simulink model "BKK7"  (Simulink 7.3)
settings: Solver=ode45  StartTime=0.0  StopTime=60  RelTol=1e-3
libraries: simulink x4
settings Model: Creator=AlexHomeLab  LastModifiedBy=Sainquake

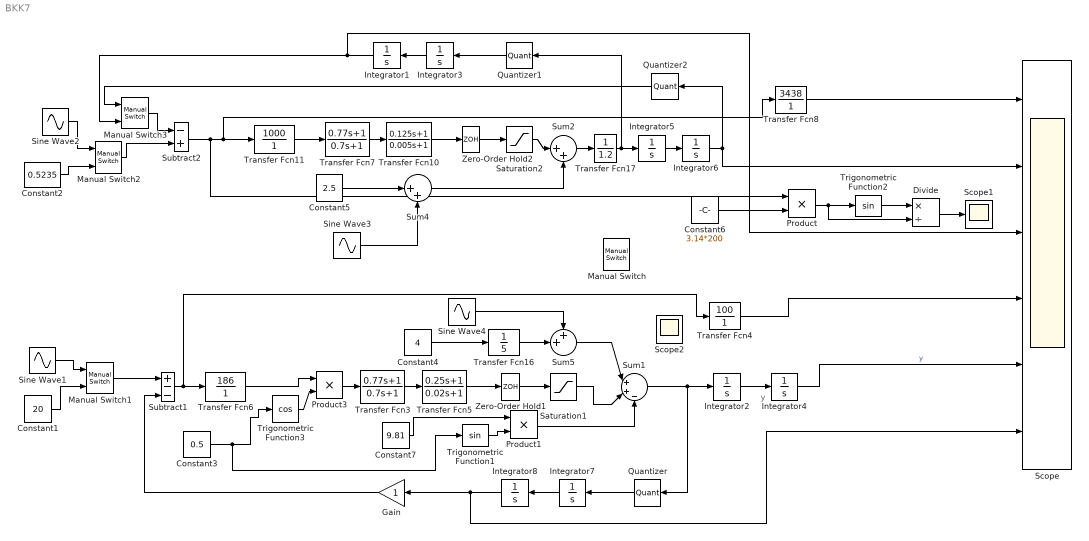
== system BKK7 ==
  note: y
  Constant1 : Constant  Value=20
  Constant2 : Constant  Value=0.5235
  Constant3 : Constant  Value=0.5
  Constant4 : Constant  Value=4
  Constant5 : Constant  Value=2.5
  Constant6 : Constant  Value=3.14*200
  Constant7 : Constant  Value=9.81
  Divide : Product  Inputs=*/  OutDataType=fixdt(1, 16)  OutScaling=2^-10
  Gain : Gain  ParameterDataType=fixdt(1, 16)  ParameterScaling=2^0  OutDataType=fixdt(1, 16)  OutScaling=2^0
  Integrator{1..8} (8 alike) : Integrator
  Manual Switch : simulink/Signal Routing/Manual Switch  SystemSampleTime=-1  sw=1  action=0  varsize=off
  Manual Switch1 : simulink/Signal Routing/Manual Switch  SystemSampleTime=-1  sw=0  action=0  varsize=off
  Manual Switch2 : simulink/Signal Routing/Manual Switch  SystemSampleTime=-1  sw=0  action=0  varsize=off
  Manual Switch3 : simulink/Signal Routing/Manual Switch  SystemSampleTime=-1  sw=0  action=0  varsize=off
  Product : Product  OutDataType=fixdt(1, 16)  OutScaling=2^0  RndMeth=Zero
  Product1 : Product  RndMeth=Zero
  Product3 : Product  RndMeth=Zero
  Quantizer : Quantizer  QuantizationInterval=0.00390625  SampleTime=1/200
  Quantizer1 : Quantizer  QuantizationInterval=0.00390625  SampleTime=1/200
  Quantizer2 : Quantizer  QuantizationInterval=0.00390625  SampleTime=1/200
  Saturation1 : Saturate  UpperLimit=17.2  LowerLimit=-17.2
  Saturation2 : Saturate  UpperLimit=20  LowerLimit=-20
  Scope : Scope  NumInputPorts=6
      settings: YMin=-45~0~-500~0~-750~0  YMax=5~60~2000~25~2000~0.7  MaxDataPoints=5000000
  Scope1 : Scope
      settings: SaveName=ScopeData2  MaxDataPoints=500000
  Scope2 : Scope
      settings: YMin=4.916  YMax=4.927  MaxDataPoints=500000
  Sine Wave1 : Sin  Amplitude=0.1  Bias=0  Frequency=0.628  Phase=0  Samples=10  SampleTime=0  Offset=0
  Sine Wave2 : Sin  Amplitude=0.1  Bias=0  Frequency=0.628  Phase=0  Samples=10  SampleTime=0  Offset=0
  Sine Wave3 : Sin  Amplitude=0.5  Bias=0  Frequency=6.28  Phase=1.57  Samples=10  SampleTime=0  Offset=0
  Sine Wave4 : Sin  Amplitude=0.3  Bias=0  Frequency=0.3  Phase=1.57  Samples=10  SampleTime=0  Offset=0
  Subtract1 : Sum  Inputs=+--
  Subtract2 : Sum  Inputs=-+
  Sum1 : Sum  Inputs=|++-
  Sum2 : Sum  Inputs=|++
  Sum4 : Sum  Inputs=|++
  Sum5 : Sum  Inputs=++|
  Transfer Fcn10 : TransferFcn  Numerator=[0.125 1]  Denominator="[0.005  1]"
  Transfer Fcn11 : TransferFcn  Numerator=1000  Denominator=[ 1 ]
  Transfer Fcn16 : TransferFcn  Denominator=[ 5 ]
  Transfer Fcn17 : TransferFcn  Denominator=[ 1.2 ]
  Transfer Fcn3 : TransferFcn  Numerator=[0.77 1]  Denominator="[0.7  1]"
  Transfer Fcn4 : TransferFcn  Numerator=[100]  Denominator=[ 1 ]
  Transfer Fcn5 : TransferFcn  Numerator=[0.25 1]  Denominator="[0.02  1]"
  Transfer Fcn6 : TransferFcn  Numerator=186  Denominator=[ 1 ]
  Transfer Fcn7 : TransferFcn  Numerator=[0.77 1]  Denominator="[0.7  1]"
  Transfer Fcn8 : TransferFcn  Numerator=[3438]  Denominator=[ 1 ]
  Trigonometric Function1 : Trigonometry
  Trigonometric Function2 : Trigonometry
  Trigonometric Function3 : Trigonometry  Operator=cos
  Zero-Order Hold1 : ZeroOrderHold  SampleTime=1/200
  Zero-Order Hold2 : ZeroOrderHold  SampleTime=1/200
  wires:
  Subtract1/1 -> Transfer Fcn6/1, Transfer Fcn4/1
  Transfer Fcn3/1 -> Transfer Fcn5/1
  Integrator2/1 -> Integrator4/1
  Constant1/1 -> Manual Switch1/2
  Product1/1 -> Sum1/3
  Sum1/1 -> Integrator2/1, Quantizer/1
  Transfer Fcn5/1 -> Zero-Order Hold1/1
  Constant4/1 -> Transfer Fcn16/1
  Sine Wave1/1 -> Manual Switch1/1
  Trigonometric Function1/1 -> Product1/2
  Constant7/1 -> Product1/1
  Trigonometric Function3/1 -> Product3/2
  Product3/1 -> Transfer Fcn3/1
  Transfer Fcn6/1 -> Product3/1
  Zero-Order Hold1/1 -> Saturation1/1
  Saturation1/1 -> Sum1/2
  Transfer Fcn16/1 -> Sum5/2
  Quantizer/1 -> Integrator7/1
  Gain/1 -> Subtract1/3
  Integrator7/1 -> Integrator8/1
  Manual Switch1/1 -> Subtract1/1
  Integrator8/1 -> Gain/1, Scope/6
  Subtract2/1 -> Transfer Fcn11/1, Transfer Fcn8/1, Product/1
  Transfer Fcn11/1 -> Transfer Fcn7/1
  Transfer Fcn7/1 -> Transfer Fcn10/1
  Integrator5/1 -> Integrator6/1
  Constant2/1 -> Manual Switch2/2
  Sine Wave2/1 -> Manual Switch2/1
  Sum2/1 -> Transfer Fcn17/1
  Transfer Fcn10/1 -> Zero-Order Hold2/1
  Sum4/1 -> Sum2/2
  Constant5/1 -> Sum4/1
  Sine Wave3/1 -> Sum4/2
  Zero-Order Hold2/1 -> Saturation2/1
  Saturation2/1 -> Sum2/1
  Manual Switch2/1 -> Subtract2/2
  Transfer Fcn8/1 -> Scope/1
  Integrator6/1 -> Quantizer2/1, Scope/2
  Manual Switch3/1 -> Subtract2/1
  Quantizer1/1 -> Integrator3/1
  Integrator3/1 -> Integrator1/1
  Integrator1/1 -> Manual Switch3/2, Scope/3
  Integrator4/1 -> Scope/5  "y"
  Transfer Fcn4/1 -> Scope/4
  Constant3/1 -> Trigonometric Function3/1, Trigonometric Function1/1
  Sum5/1 -> Sum1/1
  Sine Wave4/1 -> Sum5/1
  Transfer Fcn17/1 -> Integrator5/1, Quantizer1/1
  Quantizer2/1 -> Manual Switch3/1
  Constant6/1 -> Product/2
  Product/1 -> Trigonometric Function2/1, Divide/2
  Trigonometric Function2/1 -> Divide/1
  Divide/1 -> Scope1/1
